simulink model "z3"  (R2017b)
settings: Solver=FixedStepDiscrete  StartTime=0.0  StopTime=0  RelTol=1e-3
undefined symbols (not defined in the file or in its folder): W
libraries: CPOiS_SourcesSinks x20, CPOiS_LinearTransforms x8, CPOiS_Filters x4, CPOiS_DataManipulation_DataTypeConversion x4
settings Model: Creator=alis  LastModifiedBy=alis

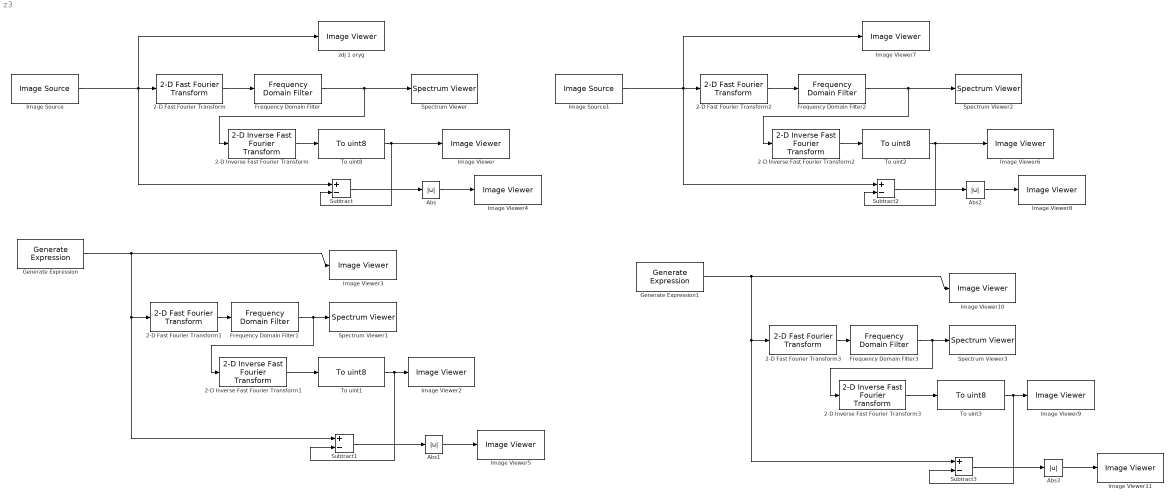
== system z3 ==
  2-D Fast Fourier Transform{,1..3} (4 alike) : CPOiS_LinearTransforms/2-D Fast Fourier Transform
      settings: SourceProductName=CPOiS - Digital image and signal processing
  2-D Inverse Fast Fourier Transform{,1..3} (4 alike) : CPOiS_LinearTransforms/2-D Inverse Fast  Fourier Transform
      settings: SourceProductName=CPOiS - Digital image and signal processing
  Abs{,1..3} (4 alike) : Abs
  Frequency Domain Filter : CPOiS_Filters/Frequency Domain Filter  filtertype=Low-pass Filter  radius=10
      settings: SourceProductName=CPOiS - Digital image and signal processing
  Frequency Domain Filter1 : CPOiS_Filters/Frequency Domain Filter  filtertype=Low-pass Filter  radius=10
      settings: SourceProductName=CPOiS - Digital image and signal processing
  Frequency Domain Filter2 : CPOiS_Filters/Frequency Domain Filter  filtertype=High-pass Filter  radius=10
      settings: SourceProductName=CPOiS - Digital image and signal processing
  Frequency Domain Filter3 : CPOiS_Filters/Frequency Domain Filter  filtertype=High-pass Filter  radius=10
      settings: SourceProductName=CPOiS - Digital image and signal processing
  Generate Expression : CPOiS_SourcesSinks/Generate Expression  Width=256  Height=256  Expression=128.*(sin(W)+1)
      settings: SourceProductName=CPOiS - Digital image and signal processing
  Generate Expression1 : CPOiS_SourcesSinks/Generate Expression  Width=256  Height=256  Expression=128.*(sin(W)+1)
      settings: SourceProductName=CPOiS - Digital image and signal processing
  Image Source : CPOiS_SourcesSinks/Image Source  FileSelection=moon.png
      settings: SourceProductName=CPOiS - Digital image and signal processing
  Image Source1 : CPOiS_SourcesSinks/Image Source  FileSelection=moon.png
      settings: SourceProductName=CPOiS - Digital image and signal processing
  Image Viewer{,2..11} (11 alike) : CPOiS_SourcesSinks/Image Viewer
      settings: SourceProductName=CPOiS - Digital image and signal processing
  Spectrum Viewer{,1..3} (4 alike) : CPOiS_SourcesSinks/Spectrum Viewer
      settings: SourceProductName=CPOiS - Digital image and signal processing
  Subtract{,1..3} (4 alike) : Sum  Inputs=+-
  To uint{1..3,8} (4 alike) : CPOiS_DataManipulation_DataTypeConversion/To uint8
      settings: SourceProductName=CPOiS - Digital image and signal processing
  zdj 1 oryg : CPOiS_SourcesSinks/Image Viewer
      settings: SourceProductName=CPOiS - Digital image and signal processing
  wires:
  Image Source/1 -> Subtract/1, zdj 1 oryg/1, 2-D Fast Fourier Transform/1
  2-D Fast Fourier Transform/1 -> Frequency Domain Filter/1
  2-D Inverse Fast Fourier Transform/1 -> To uint8/1
  2-D Inverse Fast Fourier Transform1/1 -> To uint1/1
  2-D Fast Fourier Transform1/1 -> Frequency Domain Filter1/1
  To uint8/1 -> Subtract/2, Image Viewer/1
  Subtract/1 -> Abs/1
  Abs/1 -> Image Viewer4/1
  Abs1/1 -> Image Viewer5/1
  To uint1/1 -> Subtract1/2, Image Viewer2/1
  Subtract1/1 -> Abs1/1
  Frequency Domain Filter/1 -> 2-D Inverse Fast Fourier Transform/1, Spectrum Viewer/1
  Generate Expression/1 -> Image Viewer3/1, Subtract1/1, 2-D Fast Fourier Transform1/1
  Abs2/1 -> Image Viewer8/1
  To uint2/1 -> Subtract2/2, Image Viewer6/1
  Subtract2/1 -> Abs2/1
  2-D Fast Fourier Transform2/1 -> Frequency Domain Filter2/1
  2-D Inverse Fast Fourier Transform2/1 -> To uint2/1
  Frequency Domain Filter2/1 -> 2-D Inverse Fast Fourier Transform2/1, Spectrum Viewer2/1
  Image Source1/1 -> Subtract2/1, Image Viewer7/1, 2-D Fast Fourier Transform2/1
  Frequency Domain Filter1/1 -> 2-D Inverse Fast Fourier Transform1/1, Spectrum Viewer1/1
  2-D Inverse Fast Fourier Transform3/1 -> To uint3/1
  To uint3/1 -> Subtract3/2, Image Viewer9/1
  Frequency Domain Filter3/1 -> 2-D Inverse Fast Fourier Transform3/1, Spectrum Viewer3/1
  Generate Expression1/1 -> Image Viewer10/1, Subtract3/1, 2-D Fast Fourier Transform3/1
  2-D Fast Fourier Transform3/1 -> Frequency Domain Filter3/1
  Abs3/1 -> Image Viewer11/1
  Subtract3/1 -> Abs3/1
